simulink model "RSP"  (R2023a)
settings: Solver=FixedStepDiscrete  StartTime=0.0  StopTime=1.1*pri*N_observation  FixedStep=1.220703125E-8  RelTol=1e-3  EnableMultiTasking=on
model workspace (MAT data in the model file):
  Lambda = Simulink.Parameter
  Lambda.Value = 0.1
  Lambda.DataType = 'auto'
  Lambda.Complexity = 'real'
  Lambda.Dimensions = [1 1]
  N_observation = Simulink.Parameter
  N_observation.Value = 10
  N_observation.DataType = 'auto'
  N_observation.Complexity = 'real'
  N_observation.Dimensions = [1 1]
  N_sample = Simulink.Parameter
  N_sample.Value = 8192
  N_sample.DataType = 'auto'
  N_sample.Complexity = 'real'
  N_sample.Dimensions = [1 1]
  T_sampling = Simulink.Parameter
  T_sampling.Value = Simulink.data.Expression
  T_sampling.Value.ExpressionString = "T_symbol/N_sample"
  T_sampling.DataType = 'auto'
  T_sampling.Complexity = 'real'
  T_sampling.Dimensions = -1
  T_symbol = Simulink.Parameter
  T_symbol.Value = 0.0001
  T_symbol.DataType = 'auto'
  T_symbol.Complexity = 'real'
  T_symbol.Dimensions = [1 1]
  pri = Simulink.Parameter
  pri.Value = Simulink.data.Expression
  pri.Value.ExpressionString = "(T_symbol*symbol_delay)"
  pri.DataType = 'auto'
  pri.Complexity = 'real'
  pri.Dimensions = -1
  symbol_delay = Simulink.Parameter
  symbol_delay.Value = 2
  symbol_delay.DataType = 'auto'
  symbol_delay.Complexity = 'real'
  symbol_delay.Dimensions = [1 1]
libraries: hdlsllib x4, dsphdlxfrm2 x1
(part 1 of 49)
settings Model: SimulationMode=accelerator  Creator=acer  LastModifiedBy=acer
settings SolverCC: AutoInsertRateTranBlk=on
settings OptimizationCC: BlockReduction=off  ConditionallyExecuteInputs=off
settings DebuggingCC: SingleTaskRateTransMsg=error
settings HardwareCC: ProdBitPerPointer=32  ProdBitPerSizeT=32  ProdBitPerPtrDiffT=32  ProdLargestAtomicFloat=None  ProdIntDivRoundTo=Undefined  ProdEndianess=Unspecified  ProdWordSize=32  ProdHWDeviceType=ASIC/FPGA->ASIC/FPGA  TargetBitPerPointer=64  TargetBitPerSizeT=64  TargetBitPerPtrDiffT=64  TargetLongLongMode=on  TargetIntDivRoundTo=Zero  TargetEndianess=LittleEndian  TargetWordSize=64  TargetHWDeviceType=Custom Processor->MATLAB Host Computer  ProdEqTarget=off

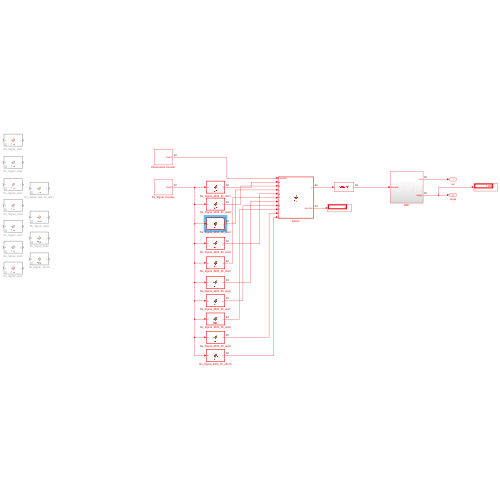
[thumbnail: Simulink's stored preview of the top-level diagram]
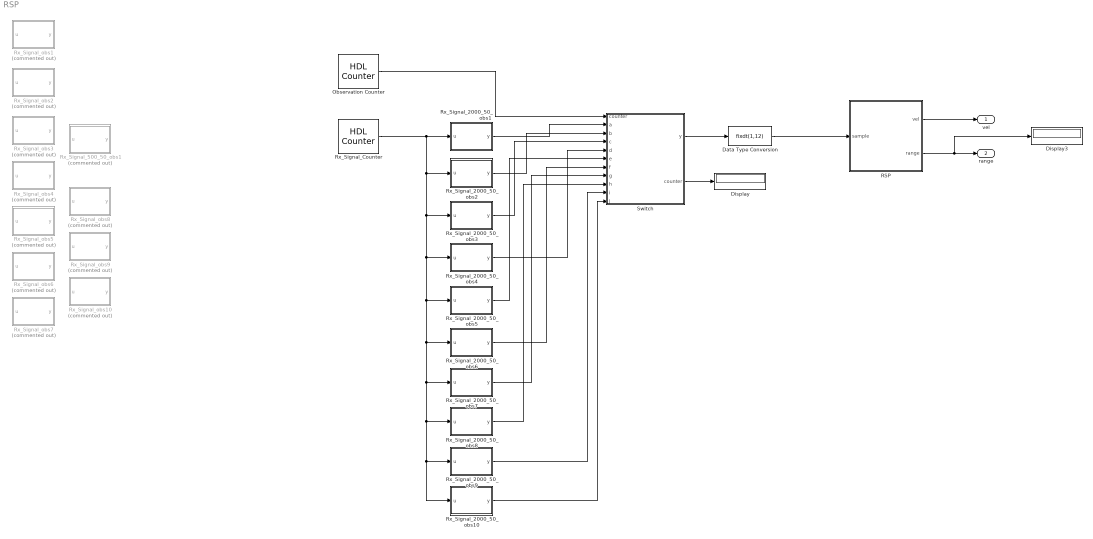
== system RSP ==
  Data Type Conversion : DataTypeConversion  OutMin=0  OutMax=1  OutDataTypeStr=fixdt(1,12)  SaturateOnIntegerOverflow=off  RndMeth=Floor
  Display : Display
  Display3 : Display
  Observation Counter : hdlsllib/Sources/HDL Counter  CountType=Count limited  CountInit=0  CountStep=1  CountMax=(N_sample * symbol_delay * N_observation) - 1  CountFromType=Initial value  CountFrom=0  CountResetPort=off  CountLoadPort=off  CountEnbPort=off  CountDirPort=off  CountHitOutputPort=off  CountDataType=Unsigned  CountWordLen=32  CountFracLen=0  CountSampTime=T_sampling
  RSP : Subsystem
  Rx_Signal_2000_50_obs1 : MATLAB Function  TreatAsAtomicUnit=on
  Rx_Signal_2000_50_obs10 : MATLAB Function  TreatAsAtomicUnit=on
  Rx_Signal_2000_50_obs2 : MATLAB Function  TreatAsAtomicUnit=on
  Rx_Signal_2000_50_obs3 : MATLAB Function  TreatAsAtomicUnit=on
  Rx_Signal_2000_50_obs4 : MATLAB Function  TreatAsAtomicUnit=on
  Rx_Signal_2000_50_obs5 : MATLAB Function  TreatAsAtomicUnit=on
  Rx_Signal_2000_50_obs6 : MATLAB Function  TreatAsAtomicUnit=on
  Rx_Signal_2000_50_obs7 : MATLAB Function  TreatAsAtomicUnit=on
  Rx_Signal_2000_50_obs8 : MATLAB Function  TreatAsAtomicUnit=on
  Rx_Signal_2000_50_obs9 : MATLAB Function  TreatAsAtomicUnit=on
  Rx_Signal_500_50_obs1 : MATLAB Function  Commented=on  TreatAsAtomicUnit=on
  Rx_Signal_Counter : hdlsllib/Sources/HDL Counter  CountType=Count limited  CountInit=0  CountStep=1  CountMax=(N_sample * symbol_delay) - 1  CountFromType=Initial value  CountFrom=0  CountResetPort=off  CountLoadPort=off  CountEnbPort=off  CountDirPort=off  CountHitOutputPort=off  CountDataType=Unsigned  CountWordLen=16  CountFracLen=0  CountSampTime=T_sampling
  Rx_Signal_obs1 : MATLAB Function  Commented=on  TreatAsAtomicUnit=on
  Rx_Signal_obs10 : MATLAB Function  Commented=on  TreatAsAtomicUnit=on
  Rx_Signal_obs2 : MATLAB Function  Commented=on  TreatAsAtomicUnit=on
  Rx_Signal_obs3 : MATLAB Function  Commented=on  TreatAsAtomicUnit=on
  Rx_Signal_obs4 : MATLAB Function  Commented=on  TreatAsAtomicUnit=on
  Rx_Signal_obs5 : MATLAB Function  Commented=on  TreatAsAtomicUnit=on
  Rx_Signal_obs6 : MATLAB Function  Commented=on  TreatAsAtomicUnit=on
  Rx_Signal_obs7 : MATLAB Function  Commented=on  TreatAsAtomicUnit=on
  Rx_Signal_obs8 : MATLAB Function  Commented=on  TreatAsAtomicUnit=on
  Rx_Signal_obs9 : MATLAB Function  Commented=on  TreatAsAtomicUnit=on
  Switch : MATLAB Function  TreatAsAtomicUnit=on
  vel : Outport  VectorParamsAs1DForOutWhenUnconnected=off
  range : Outport  Port=2  VectorParamsAs1DForOutWhenUnconnected=off
  wires:
  Data Type Conversion/1 -> RSP/1(sample)
  RSP/1(vel) -> vel/1
  RSP/2(range) -> Display3/1, range/1
  Rx_Signal_Counter/1 -> Rx_Signal_2000_50_obs1/1(u), Rx_Signal_2000_50_obs2/1(u), Rx_Signal_2000_50_obs3/1(u), Rx_Signal_2000_50_obs4/1(u), Rx_Signal_2000_50_obs5/1(u), Rx_Signal_2000_50_obs6/1(u), Rx_Signal_2000_50_obs7/1(u), Rx_Signal_2000_50_obs8/1(u), Rx_Signal_2000_50_obs9/1(u), Rx_Signal_2000_50_obs10/1(u)
  Switch/1(y) -> Data Type Conversion/1
  Switch/2(counter) -> Display/1
  Observation Counter/1 -> Switch/1("counter ")
  Rx_Signal_2000_50_obs1/1(y) -> Switch/2(a)
  Rx_Signal_2000_50_obs2/1(y) -> Switch/3(b)
  Rx_Signal_2000_50_obs3/1(y) -> Switch/4(c)
  Rx_Signal_2000_50_obs4/1(y) -> Switch/5(d)
  Rx_Signal_2000_50_obs5/1(y) -> Switch/6(e)
  Rx_Signal_2000_50_obs6/1(y) -> Switch/7(f)
  Rx_Signal_2000_50_obs7/1(y) -> Switch/8(g)
  Rx_Signal_2000_50_obs8/1(y) -> Switch/9(h)
  Rx_Signal_2000_50_obs9/1(y) -> Switch/10(i)
  Rx_Signal_2000_50_obs10/1(y) -> Switch/11(j)

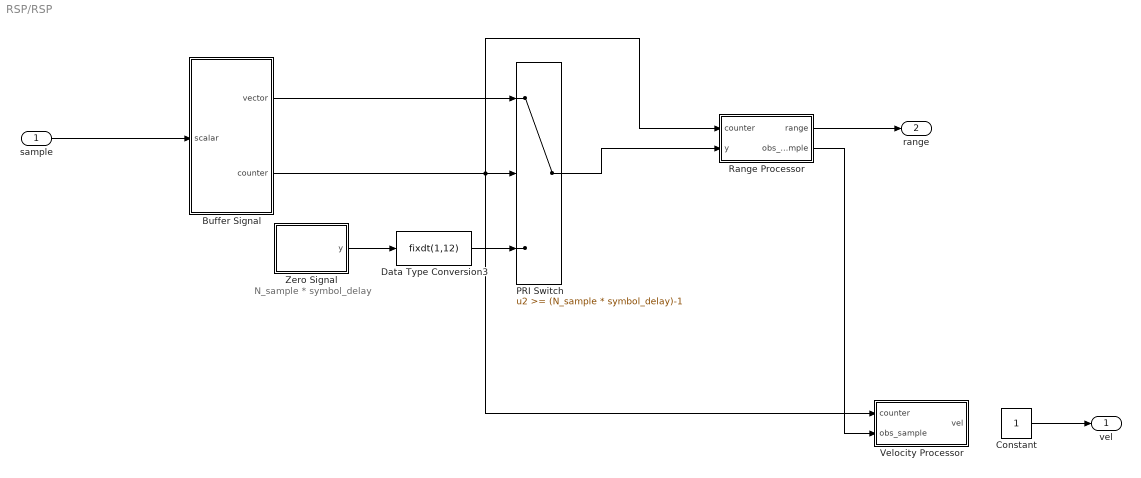
== system RSP/RSP ==
  note: N_sample * symbol_delay
  sample : Inport
  Buffer Signal : Subsystem
  Constant : Constant  OutDataTypeStr=uint8  SampleTime=-1
  Data Type Conversion3 : DataTypeConversion  OutMin=0  OutMax=1  OutDataTypeStr=fixdt(1,12)  SaturateOnIntegerOverflow=off  RndMeth=Floor
  PRI Switch : Switch  Threshold=(N_sample * symbol_delay)-1  SaturateOnIntegerOverflow=off  InputSameDT=off
  Range Processor : Subsystem
  Velocity Processor : Subsystem
  Zero Signal : MATLAB Function  TreatAsAtomicUnit=on
  vel : Outport  VectorParamsAs1DForOutWhenUnconnected=off
  range : Outport  Port=2
  wires:
  sample/1 -> Buffer Signal/1(scalar)
  Zero Signal/1(y) -> Data Type Conversion3/1
  Buffer Signal/1(vector) -> PRI Switch/1
  Data Type Conversion3/1 -> PRI Switch/3
  Buffer Signal/2(counter) -> Range Processor/1(counter), PRI Switch/2, Velocity Processor/1(counter)
  PRI Switch/1 -> Range Processor/2(y)
  Range Processor/1(range) -> range/1
  Range Processor/2(obs_sample) -> Velocity Processor/2(obs_sample)
  Constant/1 -> vel/1

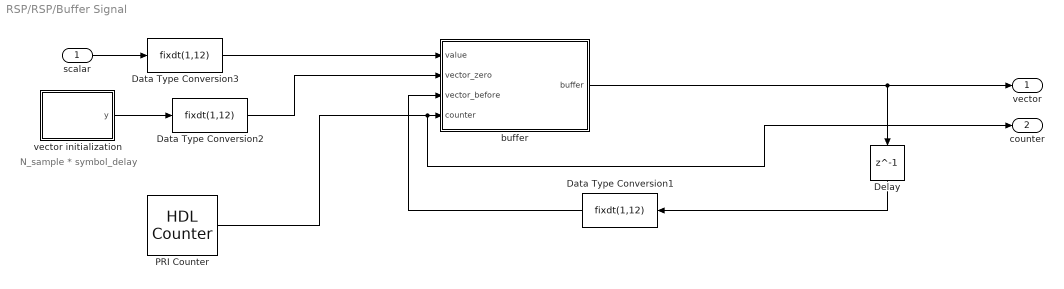
== system RSP/RSP/Buffer Signal ==
  note: N_sample * symbol_delay
  scalar : Inport
  Data Type Conversion1 : DataTypeConversion  OutMin=0  OutMax=1  OutDataTypeStr=fixdt(1,12)  SaturateOnIntegerOverflow=off  RndMeth=Floor
  Data Type Conversion2 : DataTypeConversion  OutMin=0  OutMax=1  OutDataTypeStr=fixdt(1,12)  SaturateOnIntegerOverflow=off  RndMeth=Floor
  Data Type Conversion3 : DataTypeConversion  OutMin=0  OutMax=1  OutDataTypeStr=fixdt(1,12)  SaturateOnIntegerOverflow=off  RndMeth=Floor
  Delay : Delay  DelayLength=1
  PRI Counter : hdlsllib/Sources/HDL Counter  CountType=Count limited  CountInit=0  CountStep=1  CountMax=(N_sample * symbol_delay)-1  CountFromType=Initial value  CountFrom=0  CountResetPort=off  CountLoadPort=off  CountEnbPort=off  CountDirPort=off  CountHitOutputPort=off  CountDataType=Unsigned  CountWordLen=16  CountFracLen=0  CountSampTime=T_sampling
  buffer : MATLAB Function  TreatAsAtomicUnit=on
  vector initialization : MATLAB Function  TreatAsAtomicUnit=on
  vector : Outport
  counter : Outport  Port=2  VectorParamsAs1DForOutWhenUnconnected=off
  wires:
  buffer/1(buffer) -> Delay/1, vector/1
  PRI Counter/1 -> counter/1, buffer/4(counter)
  Delay/1 -> Data Type Conversion1/1
  Data Type Conversion1/1 -> buffer/3(vector_before)
  vector initialization/1(y) -> Data Type Conversion2/1
  Data Type Conversion2/1 -> buffer/2(vector_zero)
  scalar/1 -> Data Type Conversion3/1
  Data Type Conversion3/1 -> buffer/1(value)

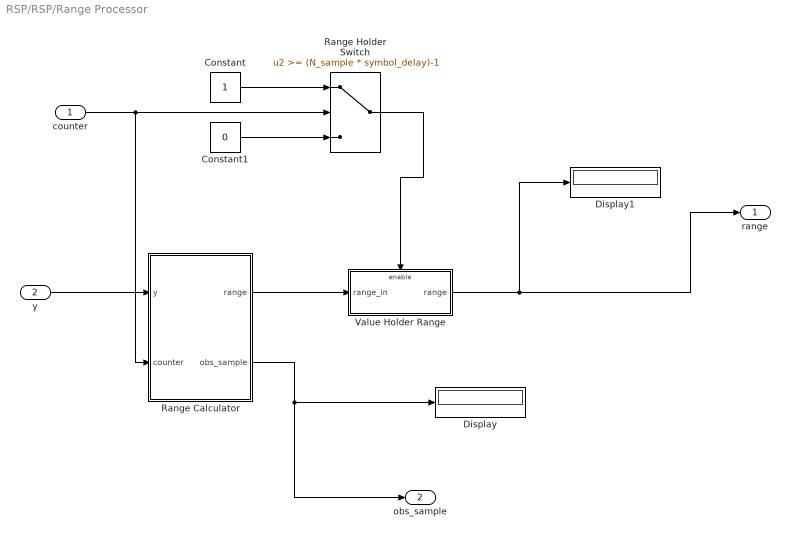
== system RSP/RSP/Range Processor ==
  counter : Inport
  y : Inport  Port=2
  Constant : Constant  OutDataTypeStr=boolean  SampleTime=-1
  Constant1 : Constant  Value=0  OutDataTypeStr=boolean  SampleTime=-1
  Display : Display
  Display1 : Display
  Range Calculator : Subsystem
  Range Holder Switch : Switch  Threshold=(N_sample * symbol_delay)-1  SaturateOnIntegerOverflow=off  InputSameDT=off
  Value Holder Range : Subsystem  TreatAsAtomicUnit=on
      settings: LibrarySourceBlock=|
      | hdlsllib/Ports &
      | Subsystems/Enabled
      | Subsystem
  range : Outport
  obs_sample : Outport  Port=2
  wires:
  counter/1 -> Range Calculator/2(counter), Range Holder Switch/2
  Range Calculator/2(obs_sample) -> obs_sample/1, Display/1
  Range Holder Switch/1 -> Value Holder Range/Enable
  Value Holder Range/1(range) -> Display1/1, range/1
  y/1 -> Range Calculator/1(y)
  Constant/1 -> Range Holder Switch/1
  Constant1/1 -> Range Holder Switch/3
  Range Calculator/1(range) -> Value Holder Range/1(range_in)

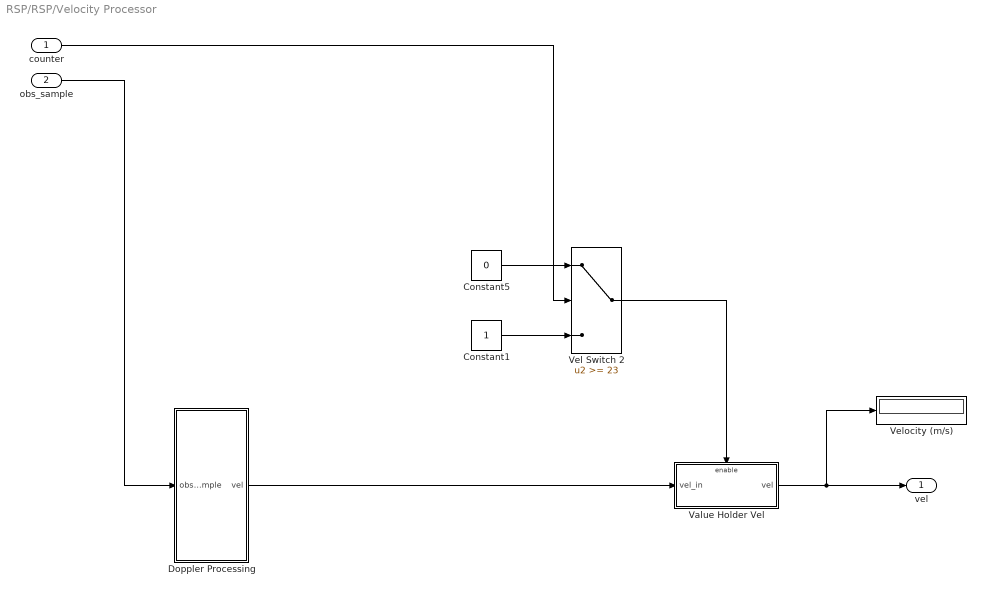
== system RSP/RSP/Velocity Processor ==
  counter : Inport
  obs_sample : Inport  Port=2
  Constant1 : Constant  OutDataTypeStr=boolean  SampleTime=-1
  Constant5 : Constant  Value=0  OutDataTypeStr=boolean  SampleTime=-1
  Doppler Processing : Subsystem
  Value Holder Vel : Subsystem  TreatAsAtomicUnit=on
      settings: LibrarySourceBlock=|
      | hdlsllib/Ports &
      | Subsystems/Enabled
      | Subsystem
  Vel Switch 2 : Switch  Threshold=23  SaturateOnIntegerOverflow=off  InputSameDT=off
  Velocity (m/s) : Display
  vel : Outport  VectorParamsAs1DForOutWhenUnconnected=off
  wires:
  obs_sample/1 -> Doppler Processing/1(obs_sample)
  Doppler Processing/1(vel) -> Value Holder Vel/1(vel_in)
  Vel Switch 2/1 -> Value Holder Vel/Enable
  Value Holder Vel/1(vel) -> vel/1, Velocity (m/s)/1
  counter/1 -> Vel Switch 2/2
  Constant1/1 -> Vel Switch 2/3
  Constant5/1 -> Vel Switch 2/1

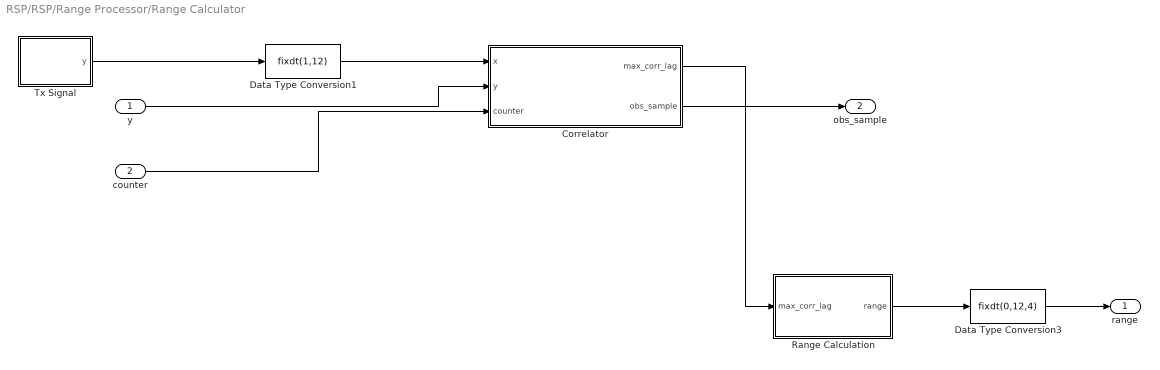
== system RSP/RSP/Range Processor/Range Calculator ==
  y : Inport
  counter : Inport  Port=2
  Correlator : MATLAB Function  TreatAsAtomicUnit=on
  Data Type Conversion1 : DataTypeConversion  OutMin=0  OutMax=1  OutDataTypeStr=fixdt(1,12)  SaturateOnIntegerOverflow=off  RndMeth=Floor
  Data Type Conversion3 : DataTypeConversion  OutMin=0  OutMax=255.9375  OutDataTypeStr=fixdt(0,12,4)  SaturateOnIntegerOverflow=off  RndMeth=Floor
  Range Calculation : Subsystem
  Tx Signal : MATLAB Function  TreatAsAtomicUnit=on
  range : Outport
  obs_sample : Outport  Port=2
  wires:
  y/1 -> Correlator/2(y)
  Data Type Conversion1/1 -> Correlator/1(x)
  Correlator/1(max_corr_lag) -> Range Calculation/1(max_corr_lag)
  Data Type Conversion3/1 -> range/1
  Range Calculation/1(range) -> Data Type Conversion3/1
  Correlator/2(obs_sample) -> obs_sample/1
  Tx Signal/1(y) -> Data Type Conversion1/1
  counter/1 -> Correlator/3(counter)

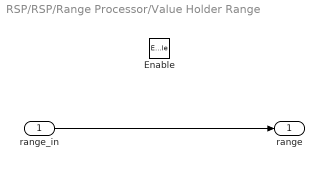
== system RSP/RSP/Range Processor/Value Holder Range ==
  range_in : Inport
  Enable : EnablePort
  range : Outport  InitialOutput=0
  wires:
  range_in/1 -> range/1

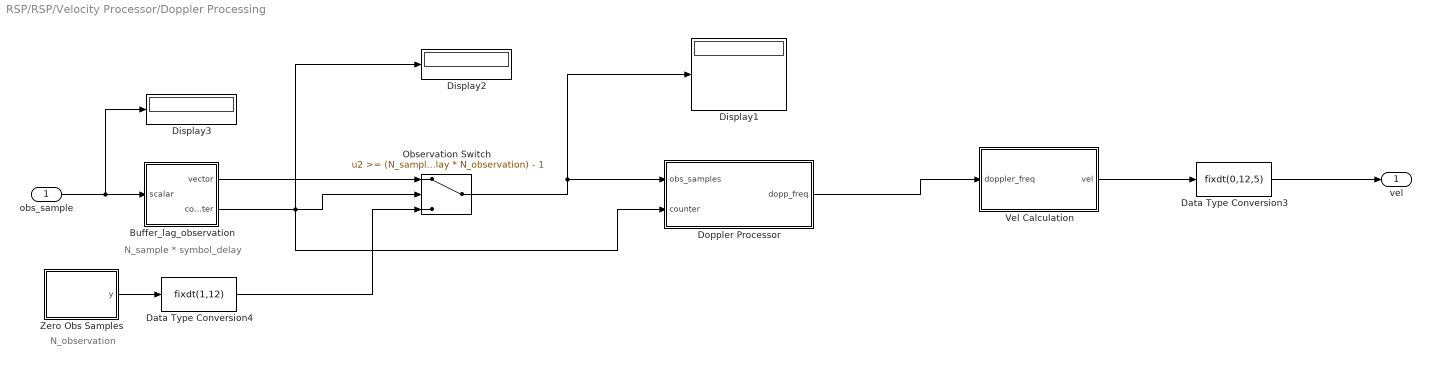
== system RSP/RSP/Velocity Processor/Doppler Processing ==
  note: N_sample * symbol_delay
  note: N_observation
  obs_sample : Inport
  Buffer_lag_observation : Subsystem
  Data Type Conversion3 : DataTypeConversion  OutMin=0  OutMax=127.969  OutDataTypeStr=fixdt(0,12,5)  SaturateOnIntegerOverflow=off  RndMeth=Floor
  Data Type Conversion4 : DataTypeConversion  OutMin=0  OutMax=1  OutDataTypeStr=fixdt(1,12)  SaturateOnIntegerOverflow=off  RndMeth=Floor
  Display1 : Display
  Display2 : Display
  Display3 : Display
  Doppler Processor : Subsystem
  Observation Switch : Switch  Threshold=(N_sample * symbol_delay * N_observation) - 1  SaturateOnIntegerOverflow=off  InputSameDT=off
  Vel Calculation : Subsystem
  Zero Obs Samples : MATLAB Function  TreatAsAtomicUnit=on
  vel : Outport
  wires:
  Data Type Conversion4/1 -> Observation Switch/3
  Zero Obs Samples/1(y) -> Data Type Conversion4/1
  Buffer_lag_observation/1(vector) -> Observation Switch/1
  obs_sample/1 -> Display3/1, Buffer_lag_observation/1(scalar)
  Buffer_lag_observation/2(counter) -> Display2/1, Observation Switch/2, Doppler Processor/2(counter)
  Data Type Conversion3/1 -> vel/1
  Vel Calculation/1(vel) -> Data Type Conversion3/1
  Doppler Processor/1(dopp_freq) -> Vel Calculation/1(doppler_freq)
  Observation Switch/1 -> Display1/1, Doppler Processor/1(obs_samples)

== system RSP/RSP/Velocity Processor/Value Holder Vel ==
  vel_in : Inport
  Enable : EnablePort
  vel : Outport  InitialOutput=0
  wires:
  vel_in/1 -> vel/1

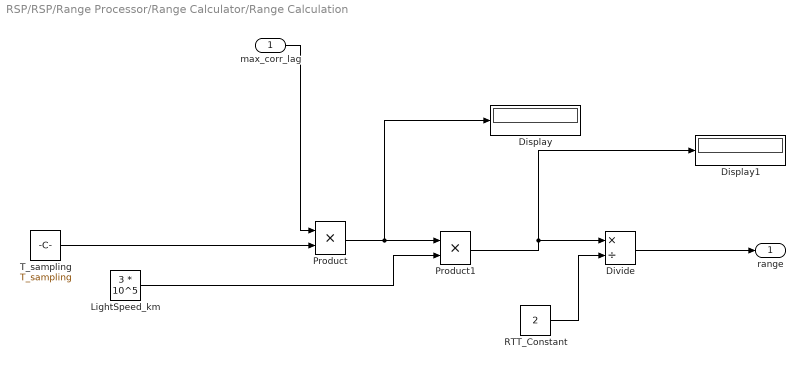
== system RSP/RSP/Range Processor/Range Calculator/Range Calculation ==
  max_corr_lag : Inport
  Display : Display
  Display1 : Display
  Divide : Product  Inputs=*/  RndMeth=Zero  SaturateOnIntegerOverflow=on
  LightSpeed_km : Constant  Value=3 * 10^5  OutDataTypeStr=fixdt(0,32,0)  SampleTime=-1
  Product : Product
  Product1 : Product
  RTT_Constant : Constant  Value=2  OutDataTypeStr=uint8  SampleTime=-1
  T_sampling : Constant  Value=T_sampling  OutDataTypeStr=fixdt(1,32,31)  SampleTime=-1
  range : Outport
  wires:
  Product/1 -> Display/1, Product1/1
  RTT_Constant/1 -> Divide/2
  T_sampling/1 -> Product/2
  Divide/1 -> range/1
  Product1/1 -> Display1/1, Divide/1
  LightSpeed_km/1 -> Product1/2
  max_corr_lag/1 -> Product/1

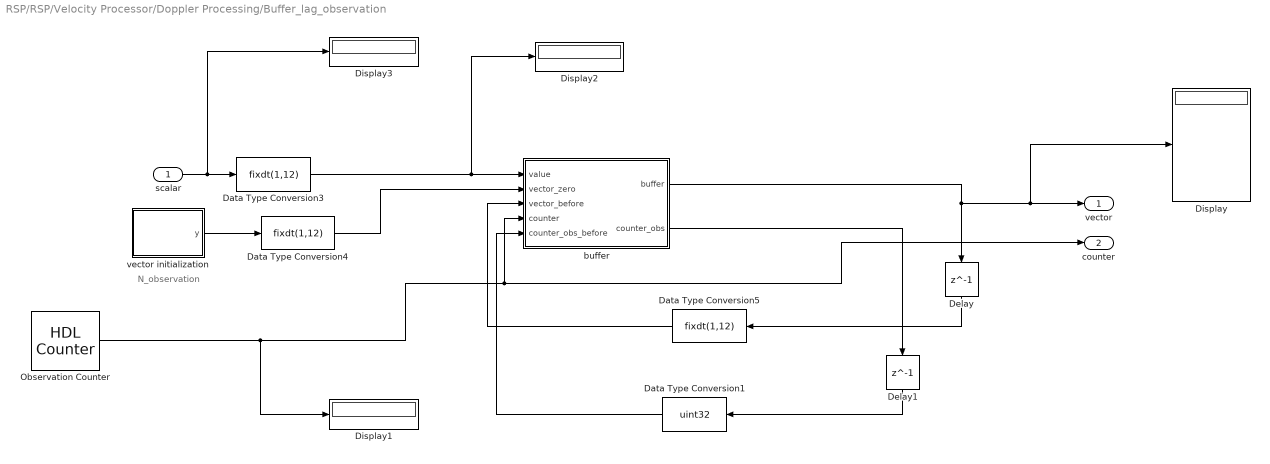
== system RSP/RSP/Velocity Processor/Doppler Processing/Buffer_lag_observation ==
  note: N_observation
  scalar : Inport
  Data Type Conversion1 : DataTypeConversion  OutMin=0  OutMax=65535  OutDataTypeStr=uint32  SaturateOnIntegerOverflow=off  RndMeth=Floor
  Data Type Conversion3 : DataTypeConversion  OutMin=0  OutMax=1  OutDataTypeStr=fixdt(1,12)  SaturateOnIntegerOverflow=off  RndMeth=Floor
  Data Type Conversion4 : DataTypeConversion  OutMin=0  OutMax=1  OutDataTypeStr=fixdt(1,12)  SaturateOnIntegerOverflow=off  RndMeth=Floor
  Data Type Conversion5 : DataTypeConversion  OutMin=0  OutMax=1  OutDataTypeStr=fixdt(1,12)  SaturateOnIntegerOverflow=off  RndMeth=Floor
  Delay : Delay  DelayLength=1
  Delay1 : Delay  DelayLength=1
  Display{,1..3} (4 alike) : Display
  Observation Counter : hdlsllib/Sources/HDL Counter  CountType=Count limited  CountInit=0  CountStep=1  CountMax=(N_sample * symbol_delay * N_observation) - 1  CountFromType=Initial value  CountFrom=0  CountResetPort=off  CountLoadPort=off  CountEnbPort=off  CountDirPort=off  CountHitOutputPort=off  CountDataType=Unsigned  CountWordLen=32  CountFracLen=0  CountSampTime=T_sampling
  buffer : MATLAB Function  TreatAsAtomicUnit=on
  vector initialization : MATLAB Function  TreatAsAtomicUnit=on
  vector : Outport
  counter : Outport  Port=2  VectorParamsAs1DForOutWhenUnconnected=off
  wires:
  buffer/1(buffer) -> Delay/1, Display/1, vector/1
  Observation Counter/1 -> Display1/1, buffer/4(counter), counter/1
  Delay/1 -> Data Type Conversion5/1
  Data Type Conversion5/1 -> buffer/3(vector_before)
  vector initialization/1(y) -> Data Type Conversion4/1
  Data Type Conversion4/1 -> buffer/2(vector_zero)
  scalar/1 -> Display3/1, Data Type Conversion3/1
  Data Type Conversion3/1 -> Display2/1, buffer/1(value)
  buffer/2(counter_obs) -> Delay1/1
  Delay1/1 -> Data Type Conversion1/1
  Data Type Conversion1/1 -> buffer/5(counter_obs_before)

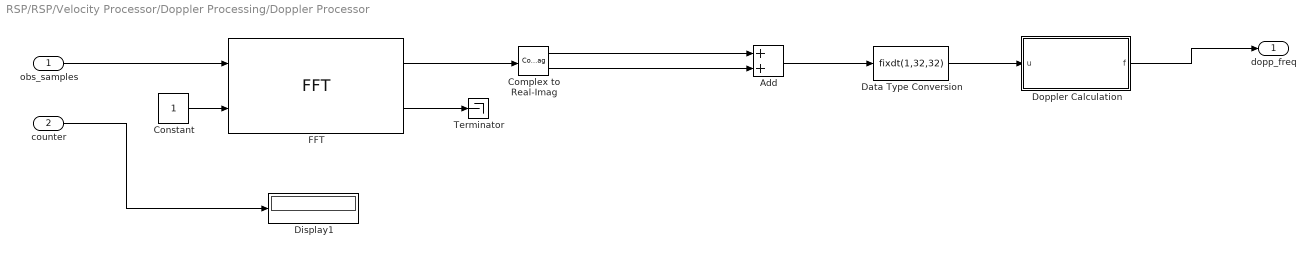
== system RSP/RSP/Velocity Processor/Doppler Processing/Doppler Processor ==
  obs_samples : Inport
  counter : Inport  Port=2
  Add : Sum
  Complex to Real-Imag : ComplexToRealImag
  Constant : Constant  OutDataTypeStr=boolean  SampleTime=-1
  Data Type Conversion : DataTypeConversion  OutDataTypeStr=fixdt(1,32,32)  SaturateOnIntegerOverflow=off  RndMeth=Floor
  Display1 : Display
  Doppler Calculation : MATLAB Function  TreatAsAtomicUnit=on
  FFT : dsphdlxfrm2/FFT  FFTLength=32  Architecture=Streaming Radix 2^2  ComplexMultiplication=Use 4 multipliers and 2 adders  BitReversedOutput=on  BitReversedInput=off  Normalize=off  SimulateUsing=Code generation  RoundingMethod=Floor  ResetInputPort=off  StartOutputPort=off  EndOutputPort=off
  Terminator : Terminator
  dopp_freq : Outport
  wires:
  Doppler Calculation/1(f) -> dopp_freq/1
  Data Type Conversion/1 -> Doppler Calculation/1(u)
  Add/1 -> Data Type Conversion/1
  counter/1 -> Display1/1
  obs_samples/1 -> FFT/1
  FFT/2 -> Terminator/1
  FFT/1 -> Complex to Real-Imag/1
  Constant/1 -> FFT/2
  Complex to Real-Imag/1 -> Add/1
  Complex to Real-Imag/2 -> Add/2

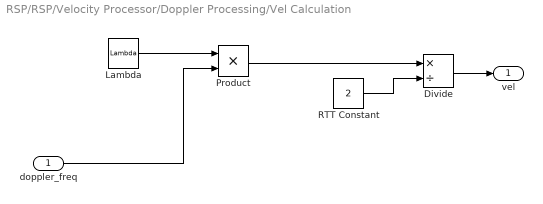
== system RSP/RSP/Velocity Processor/Doppler Processing/Vel Calculation ==
  doppler_freq : Inport
  Divide : Product  Inputs=*/  RndMeth=Zero  SaturateOnIntegerOverflow=on
  Lambda : Constant  Value=Lambda  OutDataTypeStr=fixdt(0,12,6)  SampleTime=-1
  Product : Product
  RTT Constant : Constant  Value=2  OutDataTypeStr=uint8  SampleTime=-1
  vel : Outport
  wires:
  RTT Constant/1 -> Divide/2
  Product/1 -> Divide/1
  Lambda/1 -> Product/1
  doppler_freq/1 -> Product/2
  Divide/1 -> vel/1

== matlab function RSP/Velocity Processor/Doppler Processing/Buffer_lag_observation/buffer ==
  data: value input; vector_zero input; vector_before input; counter input; buffer output; counter_obs_before input; counter_obs output
function [buffer, counter_obs] = fcn(value, vector_zero, vector_before, counter, counter_obs_before)
%#codegen

if(counter == 0)
    buffer = vector_zero;
    counter_obs = uint32(0);
elseif (mod(counter+1, 8192 * 2) == 0)
    buffer = vector_before;
    buffer(counter_obs_before+1) = value;
    counter_obs = counter_obs_before + 1;
else
    buffer = vector_before;
    counter_obs = counter_obs_before;
end

== matlab function RSP/Velocity Processor/Doppler Processing/Buffer_lag_observation/vector initialization ==
  data: y output
function y = fcn()
%#codegen

y = uint16(zeros(32,1));

== matlab function RSP/Velocity Processor/Doppler Processing/Zero Obs Samples ==
  data: y output
function y = fcn()
%#codegen

y = uint16(zeros(32,1));
